simulink model "torque"  (R2022b)
settings: Solver=VariableStepAuto  StartTime=0.0  StopTime=60  RelTol=1e-3
values from neighbouring files (symbols this model uses):
  ts = 0.05    [ModeloMotorMaxonV1.mat]
libraries: cstblocks x1, slident x1
settings Model: Creator=jorch  LastModifiedBy=jorch

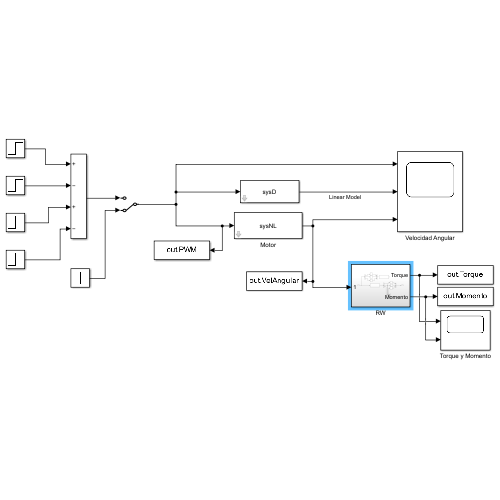
[thumbnail: Simulink's stored preview of the top-level diagram]
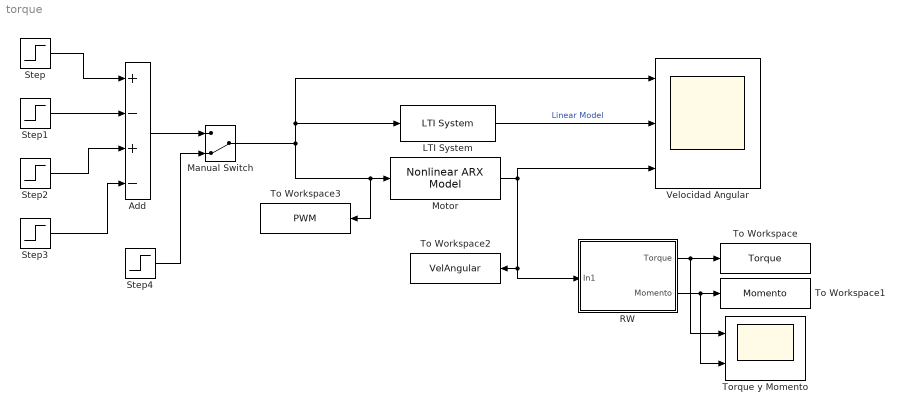
== system torque ==
  Add : Sum  Inputs=+-+-
  LTI System : cstblocks/LTI System  sys=sysD  IC=[]
  Manual Switch : ManualSwitch  CurrentSetting=0
  Motor : slident/Models/Nonlinear ARX Model  sys=sysNL  ICspec=Input and output values  X0=0  U0=0  Y0=0
  RW : Subsystem
  Step : Step  Time=10  After=80  SampleTime=ts
  Step1 : Step  Time=15  After=50  SampleTime=ts
  Step2 : Step  Time=30  After=30  SampleTime=ts
  Step3 : Step  Time=40  After=15  SampleTime=ts
  Step4 : Step  Time=30  After=99  SampleTime=ts
  To Workspace : ToWorkspace  VariableName=Torque  SampleTime=ts
  To Workspace1 : ToWorkspace  VariableName=Momento  SampleTime=ts
  To Workspace2 : ToWorkspace  VariableName=VelAngular  SampleTime=ts
  To Workspace3 : ToWorkspace  VariableName=PWM  SampleTime=ts
  Torque y Momento : Scope  NumInputPorts=2
  Velocidad Angular : Scope  NumInputPorts=3
  wires:
  Step/1 -> Add/1
  Step1/1 -> Add/2
  Step2/1 -> Add/3
  Step3/1 -> Add/4
  Manual Switch/1 -> Velocidad Angular/1, LTI System/1, Motor/1, To Workspace3/1
  LTI System/1 -> Velocidad Angular/2  "Linear Model"
  Motor/1 -> RW/1(In1), To Workspace2/1, Velocidad Angular/3
  Add/1 -> Manual Switch/1
  Step4/1 -> Manual Switch/2
  RW/1(Torque) -> Torque y Momento/1, To Workspace/1
  RW/2(Momento) -> Torque y Momento/2, To Workspace1/1

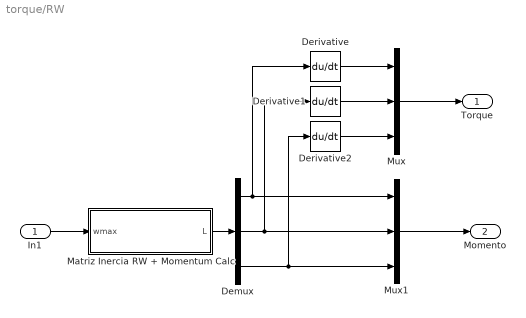
== system torque/RW ==
  In1 : Inport
  Demux : Demux  Outputs=3
  Derivative : Derivative
  Derivative1 : Derivative
  Derivative2 : Derivative
  Matriz Inercia RW + Momentum Calc : MATLAB Function  TreatAsAtomicUnit=on
  Mux : Mux  Inputs=3
  Mux1 : Mux  Inputs=3
  Torque : Outport
  Momento : Outport  Port=2
  wires:
  Demux/2 -> Mux1/2, Derivative1/1
  In1/1 -> Matriz Inercia RW + Momentum Calc/1(wmax)
  Matriz Inercia RW + Momentum Calc/1(L) -> Demux/1
  Derivative1/1 -> Mux/2
  Demux/3 -> Mux1/3, Derivative2/1
  Demux/1 -> Mux1/1, Derivative/1
  Derivative/1 -> Mux/1
  Derivative2/1 -> Mux/3
  Mux1/1 -> Momento/1
  Mux/1 -> Torque/1

== matlab function torque/RW/Matriz Inercia RW + Momentum Calc ==
  data: wmax input; L output
function L = fcn(wmax)

J_inox = [20455 0 0; 0 28389 0; 0 0 20455];

J_inox = J_inox*1E-9; % To kg m^2

L_ino = wmax*J_inox;

L = [L_ino(1,1);L_ino(2,2);L_ino(3,3)];
